simulink model "simulink_for_arduino_mealy"  (R2019b)
settings: Solver=VariableStepAuto  StartTime=0.0  StopTime=inf  FixedStep=5000  RelTol=1e-3  EnableMultiTasking=on
libraries: arduinolib x9, simulink x6
settings Model: SILPILModeSetting=veronly  ExtModeTrigDuration=2  Creator=Ahmed Zaghloul  LastModifiedBy=Ahmed Zaghloul
settings OptimizationCC: EnhancedBackFolding=on  PassReuseOutputArgsAs=Individual arguments  ZeroExternalMemoryAtStartup=off  ZeroInternalMemoryAtStartup=off  MaxStackSize=64  OptimizeBlockOrder=speed  DifferentSizesBufferReuse=on  OptimizationCustomize=off  EfficientTunableParamExpr=on
settings DebuggingCC: ParameterTunabilityLossMsg=error
settings HardwareCC: ProdBitPerInt=16  ProdBitPerPointer=16  ProdBitPerSizeT=16  ProdBitPerPtrDiffT=16  ProdLargestAtomicFloat=None  ProdWordSize=8  ProdHWDeviceType=Atmel->AVR
settings SFSimCC: MATLABDynamicMemAlloc=off
settings RTWCC: SystemTargetFile=ert.tlc  HardwareBoard=Arduino Uno  TLCOptions=-aInlineSetEventsForThisBaseRateFcn=TLC_FALSE -aSuppressMultiTaskScheduler=TLC_FALSE -aRateBasedStepFcn=1  TemplateMakefile=ert_default_tmf  Toolchain=Arduino AVR  BuildConfiguration=Faster Runs
settings CodeAppCC: ForceParamTrailComments=on  IgnoreCustomStorageClasses=off  OperatorAnnotations=on  SimulinkDataObjDesc=on  SFDataObjDesc=on  InsertBlockDesc=on
settings ERTTargetCC: SupportContinuousTime=on  SupportVariableSizeSignals=on  ExtModeStaticAllocSize=250

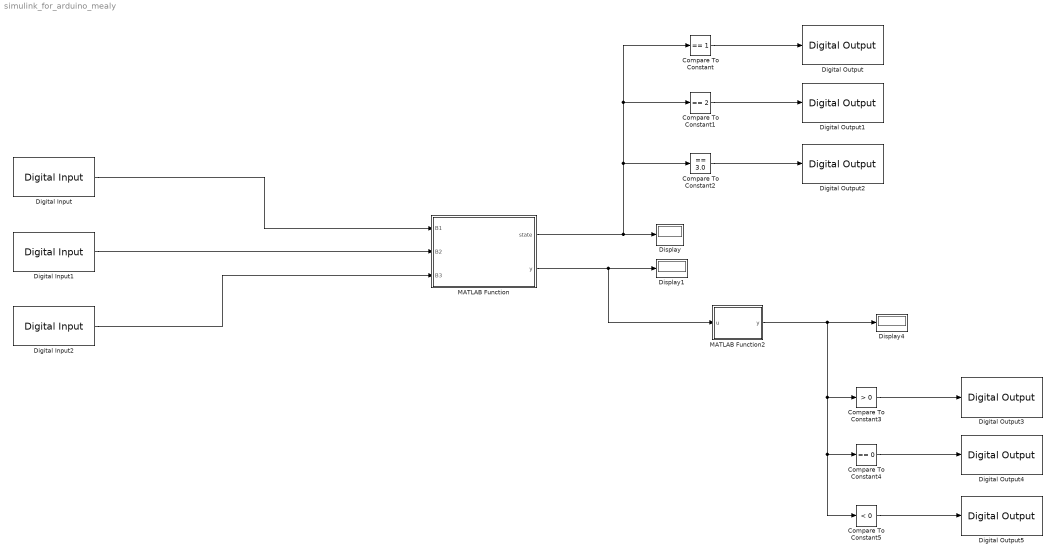
== system simulink_for_arduino_mealy ==
  Compare To Constant : simulink/Logic and Bit Operations/Compare To Constant  relop===  const=1  OutDataTypeStr=boolean
  Compare To Constant1 : simulink/Logic and Bit Operations/Compare To Constant  relop===  const=2  OutDataTypeStr=boolean
  Compare To Constant2 : simulink/Logic and Bit Operations/Compare To Constant  relop===  const=3.0  OutDataTypeStr=boolean
  Compare To Constant3 : simulink/Logic and Bit Operations/Compare To Constant  relop=>  const=0  OutDataTypeStr=boolean
  Compare To Constant4 : simulink/Logic and Bit Operations/Compare To Constant  relop===  const=0  OutDataTypeStr=boolean
  Compare To Constant5 : simulink/Logic and Bit Operations/Compare To Constant  relop=<  const=0  OutDataTypeStr=boolean
  Digital Input : arduinolib/Digital Input  pinNumber=10  mode=Default  Direction=input  SampleTime=1  blockPlatform=arduino
  Digital Input1 : arduinolib/Digital Input  pinNumber=9  mode=Default  Direction=input  SampleTime=1  blockPlatform=arduino
  Digital Input2 : arduinolib/Digital Input  pinNumber=8  mode=Default  Direction=input  SampleTime=1  blockPlatform=arduino
  Digital Output : arduinolib/Digital Output  pinNumber=2  Direction=output  blockPlatform=arduino
  Digital Output1 : arduinolib/Digital Output  pinNumber=3  Direction=output  blockPlatform=arduino
  Digital Output2 : arduinolib/Digital Output  pinNumber=4  Direction=output  blockPlatform=arduino
  Digital Output3 : arduinolib/Digital Output  pinNumber=7  Direction=output  blockPlatform=arduino
  Digital Output4 : arduinolib/Digital Output  pinNumber=6  Direction=output  blockPlatform=arduino
  Digital Output5 : arduinolib/Digital Output  pinNumber=5  Direction=output  blockPlatform=arduino
  Display : Display
  Display1 : Display
  Display4 : Display
  MATLAB Function : MATLAB Function  TreatAsAtomicUnit=on
  MATLAB Function2 : MATLAB Function  TreatAsAtomicUnit=on
  wires:
  MATLAB Function2/1(y) -> Compare To Constant5/1, Compare To Constant4/1, Compare To Constant3/1, Display4/1
  Compare To Constant/1 -> Digital Output/1
  Compare To Constant1/1 -> Digital Output1/1
  Compare To Constant2/1 -> Digital Output2/1
  Compare To Constant5/1 -> Digital Output5/1
  Compare To Constant4/1 -> Digital Output4/1
  Compare To Constant3/1 -> Digital Output3/1
  Digital Input/1 -> MATLAB Function/1(B1)
  Digital Input1/1 -> MATLAB Function/2(B2)
  Digital Input2/1 -> MATLAB Function/3(B3)
  MATLAB Function/1(state) -> Compare To Constant2/1, Compare To Constant1/1, Compare To Constant/1, Display/1
  MATLAB Function/2(y) -> MATLAB Function2/1(u), Display1/1

== matlab function simulink_for_arduino_mealy/MATLAB Function ==
  data: state output; B1 input; y output; B2 input; B3 input
function [state,y] = fcn(B1,B2,B3)
persistent current_state
if(isempty(current_state))
    current_state = 1;
end
switch current_state
    case 1
        if(B2)
            current_state = 2;
            y = "u1";
        elseif(B3)
            current_state = 3;
            y = "u2";
        else
            current_state = 1;
            y = "s";
        end
    case 2
        if(B1)
            current_state = 1;
            y = "d1";
        elseif(B3)
            current_state = 3;
            y = "u1";
        else
            current_state = 2;
            y = "s";
        end
    otherwise
        if(B1)
            current_state = 1;
            y = "d2";
        elseif(B2)
            current_state = 2;
            y = "d1";
        else
            current_state = 3;
            y = "s";
        end
end
state = current_state;
pause(0.3)
end

== matlab function simulink_for_arduino_mealy/MATLAB Function2 ==
  data: u input; y output
function y = fcn(u)
if u == "s"
    y = 0;
elseif u == "u1"
    y = 1;
elseif u == "u2"
    y = 2;
elseif u == "d1"
    y = -1;
else
    y = -2;
end
